simulink model "LC_VSI_filter"  (R2017b)
settings: Solver=ode45  StartTime=0.0  StopTime=1  RelTol=1e-3  EnableMultiTasking=on
values from neighbouring files (symbols this model uses):
  A = [-R/L -1/L; 1/C 0]    [load_sys.m]
  B = [Vcc/L; 0]    [load_sys.m]
  C = [1 0]    [load_sys.m]    (also in params.m = 2.5e-05)
  C_obsv = T_y\C_obsv*T_x    [build_obsv.m]    (also in delays_obsv.m = [C_obsv, zeros(p, m*n_d)]; noise_.m = [C_obsv zeros(p, 2)])
  C_ww = blkdiag(C_ww, C_w)    [noise_.m]
  fa = 20000    [load_sys.m]    (also in params.m = 1/Ta)
  Kp = dlqr(Phi_ctrb, Gamma_ctrb, Q, R)    [build_ctrb.m]
  L = dlqe(Phi_obsv, Psi, C_obsv, Rw, Rv)    [build_obsv.m]    (also in params.m = 0.01)
  noises = struct('')    [noise_.m]
  Psi = zeros(n, 1)    [build_obsv.m]
  T_u = 1    [build_obsv.m]
  T_x = blkdiag(T_x, T_ww)    [build_obsv.m]
  T_y = 1/100    (= 0.01)    [build_obsv.m]
  Ta = 1/fa    (= 5e-05)    [load_sys.m]    (also in params.m = ta_scaler*t_s)
  Vcc = 40    [params.m]
undefined symbols (not defined in the file or in its folder): Gamma_obsv, Phi_obsv
settings Model: Creator=brunopeixoto  LastModifiedBy=Lucas
settings DataIOCC: LimitDataPoints=on  SaveFormat=Array
settings OptimizationCC: LifeSpan=inf
settings DebuggingCC: SFUnexpectedBacktrackingDiag=warning  SFNoUnconditionalDefaultTransitionDiag=warning  SFExecutionAtInitializationDiag=none
settings HardwareCC: ProdBitPerPointer=32  ProdBitPerSizeT=32  ProdBitPerPtrDiffT=32  ProdLargestAtomicFloat=None  ProdIntDivRoundTo=Undefined  ProdEndianess=Unspecified  ProdWordSize=32  ProdHWDeviceType=32-bit Generic
settings ModelReferenceCC: PropagateSignalLabelsOutOfModel=off
settings CodeAppCC: StateflowObjectComments=on
settings GRTTargetCC: TargetLangStandard=C89/C90 (ANSI)  GeneratePreprocessorConditionals=Disable all
settings ConfigComp: CovMetricSettings=dw  CovHtmlReporting=on  CovSaveCumulativeToWorkspaceVar=on  CovSaveSingleToWorkspaceVar=on  CovExternalEMLEnable=off

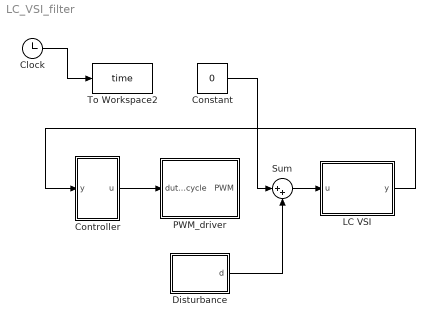
== system LC_VSI_filter ==
  Clock : Clock
  Constant : Constant  Value=0
  Controller : Subsystem
  Disturbance : Subsystem
  LC VSI : Subsystem
  PWM_driver : Subsystem
  Sum : Sum  Inputs=|++
  To Workspace2 : ToWorkspace  VariableName=time  SampleTime=Ta
      settings: Save2DSignal=2-D array (concatenate along first dimension)
  wires:
  LC VSI/1(y) -> Controller/1(y)
  Disturbance/1(d) -> Sum/2
  Controller/1(u) -> PWM_driver/1(duty_cycle)
  Constant/1 -> Sum/1
  Sum/1 -> LC VSI/1(u)
  Clock/1 -> To Workspace2/1

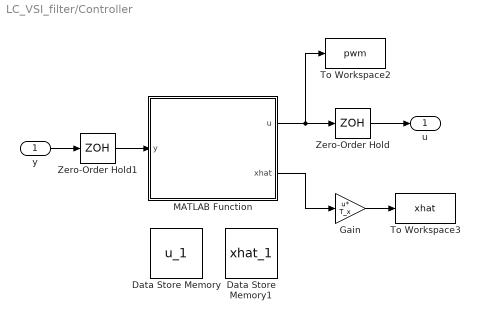
== system LC_VSI_filter/Controller ==
  y : Inport
  Data Store Memory : DataStoreMemory  DataStoreName=u_1  ReadBeforeWriteMsg=warning  WriteAfterWriteMsg=warning  WriteAfterReadMsg=warning  ShowAdditionalParam=off  OutDataTypeStr=double
  Data Store Memory1 : DataStoreMemory  DataStoreName=xhat_1  WriteAfterWriteMsg=warning  WriteAfterReadMsg=warning  InitialValue=xhat0  ShowAdditionalParam=off  OutDataTypeStr=double
  Gain : Gain  Gain=T_x  Multiplication=Matrix(u*K)
  MATLAB Function : MATLAB Function  TreatAsAtomicUnit=on
  To Workspace2 : ToWorkspace  VariableName=pwm  SampleTime=Ta
      settings: Save2DSignal=2-D array (concatenate along first dimension)
  To Workspace3 : ToWorkspace  VariableName=xhat  SampleTime=Ta
      settings: Save2DSignal=2-D array (concatenate along first dimension)
  Zero-Order Hold : ZeroOrderHold  SampleTime=Ta
  Zero-Order Hold1 : ZeroOrderHold  SampleTime=Ta
  u : Outport
  wires:
  Zero-Order Hold/1 -> u/1
  MATLAB Function/1(u) -> To Workspace2/1, Zero-Order Hold/1
  y/1 -> Zero-Order Hold1/1
  Zero-Order Hold1/1 -> MATLAB Function/1(y)
  Gain/1 -> To Workspace3/1
  MATLAB Function/2(xhat) -> Gain/1

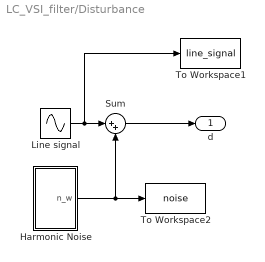
== system LC_VSI_filter/Disturbance ==
  Harmonic Noise : Subsystem
  Line signal : Sin  Amplitude=noises.('w_1').A  Frequency=noises.('w_1').w  Phase=noises.('w_1').phi  SampleTime=0
  Sum : Sum  Inputs=|++
  To Workspace1 : ToWorkspace  VariableName=line_signal  SampleTime=Ta
      settings: Save2DSignal=2-D array (concatenate along first dimension)
  To Workspace2 : ToWorkspace  VariableName=noise  SampleTime=Ta
      settings: Save2DSignal=2-D array (concatenate along first dimension)
  d : Outport
  wires:
  Harmonic Noise/1(n_w) -> Sum/2, To Workspace2/1
  Line signal/1 -> To Workspace1/1, Sum/1
  Sum/1 -> d/1

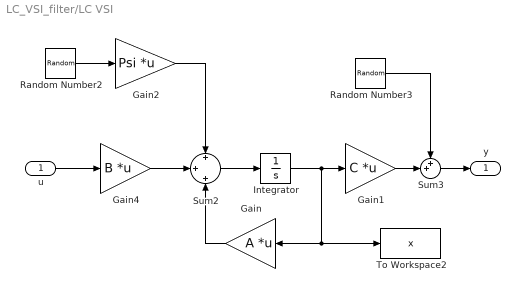
== system LC_VSI_filter/LC VSI ==
  u : Inport
  Gain : Gain  Gain=A  Multiplication=Matrix(K*u) (u vector)
  Gain1 : Gain  Gain=C  Multiplication=Matrix(K*u) (u vector)
  Gain2 : Gain  Gain=Psi  Multiplication=Matrix(K*u) (u vector)
  Gain4 : Gain  Gain=B  Multiplication=Matrix(K*u) (u vector)
  Integrator : Integrator  InitialCondition=10*[rand(), rand()]
  Random Number2 : RandomNumber  SampleTime=Ta
  Random Number3 : RandomNumber  SampleTime=Ta
  Sum2 : Sum  Inputs=+|+|+
  Sum3 : Sum  Inputs=++|
  To Workspace2 : ToWorkspace  VariableName=x  SampleTime=Ta
      settings: Save2DSignal=2-D array (concatenate along first dimension)
  y : Outport
  wires:
  Gain4/1 -> Sum2/2
  Gain/1 -> Sum2/3
  Gain1/1 -> Sum3/2
  Sum3/1 -> y/1
  u/1 -> Gain4/1
  Sum2/1 -> Integrator/1
  Gain2/1 -> Sum2/1
  Random Number3/1 -> Sum3/1
  Random Number2/1 -> Gain2/1
  Integrator/1 -> Gain1/1, To Workspace2/1, Gain/1

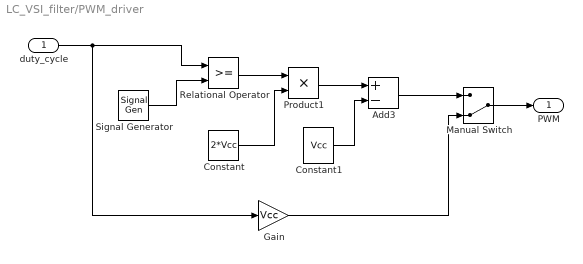
== system LC_VSI_filter/PWM_driver ==
  duty_cycle : Inport
  Add3 : Sum  Inputs=+-
  Constant : Constant  Value=2*Vcc
  Constant1 : Constant  Value=Vcc
  Gain : Gain  Gain=Vcc
  Manual Switch : ManualSwitch  CurrentSetting=0
  Product1 : Product
  Relational Operator : RelationalOperator  OutDataTypeStr=boolean  RndMeth=Nearest
  Signal Generator : SignalGenerator  WaveForm=sawtooth  Frequency=fa
  PWM : Outport
  wires:
  duty_cycle/1 -> Gain/1, Relational Operator/1
  Signal Generator/1 -> Relational Operator/2
  Product1/1 -> Add3/1
  Constant1/1 -> Add3/2
  Constant/1 -> Product1/2
  Relational Operator/1 -> Product1/1
  Manual Switch/1 -> PWM/1
  Add3/1 -> Manual Switch/1
  Gain/1 -> Manual Switch/2

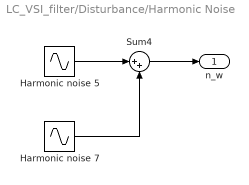
== system LC_VSI_filter/Disturbance/Harmonic Noise ==
  Harmonic noise 5 : Sin  Amplitude=noises.('w_5').A  Frequency=noises.('w_5').w  Phase=noises.('w_5').phi  SampleTime=0
  Harmonic noise 7 : Sin  Amplitude=noises.('w_7').A  Frequency=noises.('w_7').w  Phase=noises.('w_7').phi  SampleTime=0
  Sum4 : Sum  Inputs=|++
  n_w : Outport
  wires:
  Harmonic noise 7/1 -> Sum4/2
  Harmonic noise 5/1 -> Sum4/1
  Sum4/1 -> n_w/1

== matlab function LC_VSI_filter/Controller/MATLAB Function ==
  data: u output size=1; y input; Phi_obsv parameter; Gamma_obsv parameter; C_obsv parameter; L parameter; Kp parameter; xhat_1 data_store_memory; u_1 data_store_memory; C_ww parameter; xhat output; T_y parameter; T_x parameter; T_u parameter
function [u, xhat] = control(y, Phi_obsv, Gamma_obsv, C_obsv, ...
                             L, Kp, C_ww, T_y, T_x, T_u)
    global u_1 xhat_1;
    
    y = T_y*y;
    
    % Augmented noise predictor
    xbar = Phi_obsv*xhat_1 + Gamma_obsv*u_1;
    xhat = xbar + L*(y - C_obsv*xbar);
       
    xtilde = xhat(1:2);
    wtilde = C_ww*xhat(3:end);
    
     line_tilde = wtilde(1);
     noise_tilde = sum(wtilde(2:end));
    
    % Reference tracking and noise compensationw
    u = -Kp*xtilde;
       
    % Save previous value
    u_1 = u;
    xhat_1 = xhat;

    xhat = T_x*xhat;
    u = T_u*u;
end
